simulink model "LinSys"  (R2015b)
settings: Solver=VariableStepAuto  StartTime=0.0  StopTime=Simulation_Time  RelTol=1e-3
values from neighbouring files (symbols this model uses):
  A = [0 1 0 0; 0 976 0 0; 0 0 0 1; 0 0 0 0]    [LinABCD.m]
  B = [0 0; 0 12.6480816; 0 0; -33.345933008 0.506871743]    [LinABCD.m]
  C = [0 488 0 0;0 0 0 0]    [LinABCD.m]
  D = [6.3240 0;16.6729 -0.021648]    [LinABCD.m]
  Simulation_step = 0.1    [LinABCD.m]
undefined symbols (not defined in the file or in its folder): x0
settings Model: Creator=dmartin_a  LastModifiedBy=dmartin_a

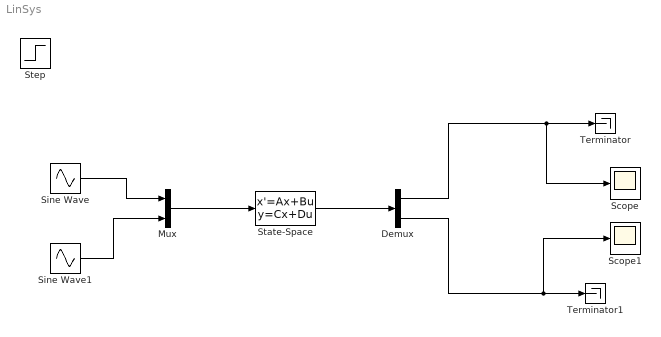
== system LinSys ==
  Demux : Demux  Outputs=2
  Mux : Mux  Inputs=2
  Scope : Scope
  Scope1 : Scope
  Sine Wave : Sin  SampleTime=0
  Sine Wave1 : Sin  SampleTime=0
  State-Space : StateSpace  A=A  B=B  C=C  D=D  X0=x0
  Step : Step  SampleTime=Simulation_step
  Terminator : Terminator
  Terminator1 : Terminator
  wires:
  Mux/1 -> State-Space/1
  State-Space/1 -> Demux/1
  Sine Wave1/1 -> Mux/2
  Demux/2 -> Terminator1/1, Scope1/1
  Demux/1 -> Terminator/1, Scope/1
  Sine Wave/1 -> Mux/1
